simulink model "ad_blue_level"  (R2018a)
settings: Solver=FixedStepAuto  StartTime=0.0  StopTime=10.0  FixedStep=1  RelTol=1e-3
undefined symbols (not defined in the file or in its folder): Ad_blue_level
libraries: simulink x3
settings Model: DataDictionary=output7_data.sldd  Creator=Home  LastModifiedBy=Home

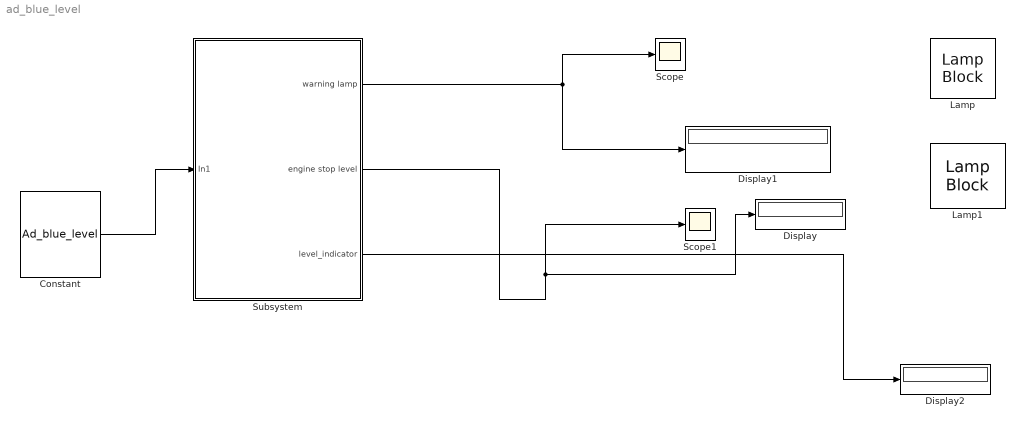
== system ad_blue_level ==
  Constant : Constant  Value=Ad_blue_level
  Display : Display
  Display1 : Display
  Display2 : Display
  Lamp : LampBlock  WebBlockId=26  LabelPosition=Bottom
  Lamp1 : LampBlock  WebBlockId=27
  Scope : Scope
  Scope1 : Scope
  Subsystem : Subsystem
  wires:
  Subsystem/1(warning lamp) -> Display1/1, Scope/1
  Subsystem/2(engine stop level) -> Scope1/1, Display/1
  Constant/1 -> Subsystem/1(In1)
  Subsystem/3("level_indicator ") -> Display2/1

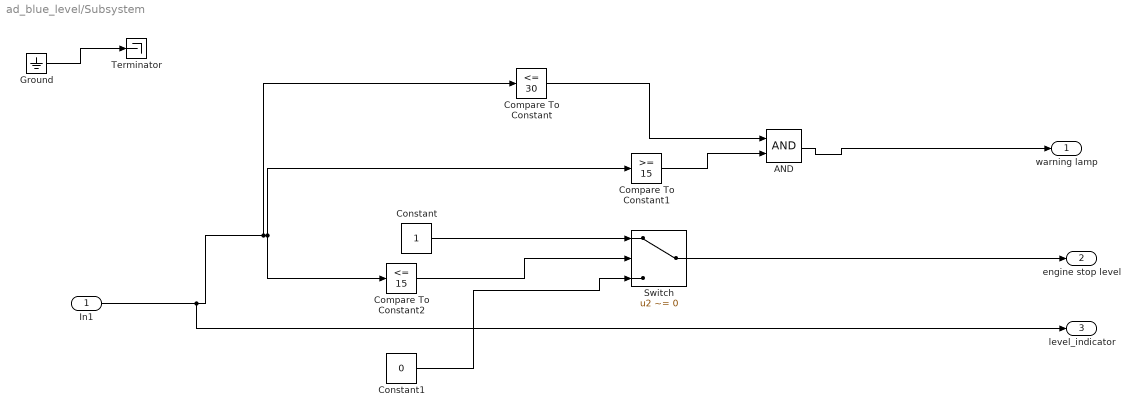
== system ad_blue_level/Subsystem ==
  In1 : Inport
  AND : Logic  AllPortsSameDT=off  OutDataTypeStr=boolean
  Compare To Constant : simulink/Logic and Bit Operations/Compare To Constant  relop=<=  const=30  OutDataTypeStr=boolean
  Compare To Constant1 : simulink/Logic and Bit Operations/Compare To Constant  relop=>=  const=15  OutDataTypeStr=boolean
  Compare To Constant2 : simulink/Logic and Bit Operations/Compare To Constant  relop=<=  const=15  OutDataTypeStr=boolean
  Constant : Constant
  Constant1 : Constant  Value=0
  Ground : Ground
  Switch : Switch  Criteria=u2 ~= 0
  Terminator : Terminator
  warning lamp : Outport
  engine stop level : Outport  Port=2
  "level_indicator " : Outport  Port=3
  wires:
  Ground/1 -> Terminator/1
  Compare To Constant/1 -> AND/1
  Compare To Constant1/1 -> AND/2
  Compare To Constant2/1 -> Switch/2
  Constant/1 -> Switch/1
  Constant1/1 -> Switch/3
  AND/1 -> warning lamp/1
  Switch/1 -> engine stop level/1
  In1/1 -> "level_indicator "/1, Compare To Constant1/1, Compare To Constant2/1, Compare To Constant/1
